simulink model "revysenal"  (R2015a)
settings: Solver=ode45  SolverMode=MultiTasking  StartTime=0.0  StopTime=(N-1)/Fs  MaxStep=1/Fs  MinStep=1/Fs  RelTol=1e-3  AbsTol=1/Fs
undefined symbols (not defined in the file): Fs
settings Model: Creator=Javi  LastModifiedBy=Javi
settings SolverCC: InitialStep=1/Fs

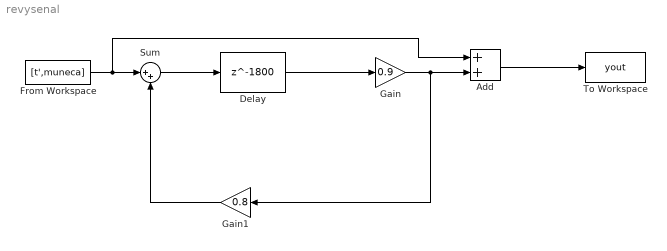
== system revysenal ==
  Add : Sum
  Delay : Delay  DelayLength=1800  SampleTime=1/Fs
  From Workspace : FromWorkspace  VariableName=[t',muneca]  SampleTime=1/Fs
  Gain : Gain  Gain=0.9
  Gain1 : Gain  Gain=0.8
  Sum : Sum  Inputs=|++  OutMin=0.0  OutMax=1.0
  To Workspace : ToWorkspace  VariableName=yout  SaveFormat=Timeseries  SampleTime=1/Fs
      settings: MaxDataPoints=N
  wires:
  Delay/1 -> Gain/1
  Gain/1 -> Gain1/1, Add/2
  From Workspace/1 -> Add/1, Sum/1
  Sum/1 -> Delay/1
  Gain1/1 -> Sum/2
  Add/1 -> To Workspace/1
